simulink model "CartesianImpedanceCtrlForUse"  (R2024a)
settings: Solver=ode45  StartTime=0.0  StopTime=tEnd+7  RelTol=1e-3
values from neighbouring files (symbols this model uses):
  Kf_gain = 100    [helperDesignImpedanceControl.m]
  neuromeka = importrobot(robotFile, DataFormat="column")    [helperDesignImpedanceControl.m]
  objectPos = 0.2    [helperDesignImpedanceControl.m]
  p_surface = [-0.30; -0.20; 0.35]    [helperDesignImpedanceControl.m]
  q_init = q_nmpc    [helperDesignImpedanceControl.m]
  tEnd = 5    [helperDesignImpedanceControl.m]
  Ts = 0.001    [helperDesignImpedanceControl.m]
  tStart = 0.5    [helperDesignImpedanceControl.m]
  use_force_feedback = 1    [helperDesignImpedanceControl.m]
undefined symbols (not defined in the file or in its folder): X, Y, Z
libraries: sm_lib x88, nesl_utility x54, matrix_library x4, robotcorelib x2, robotmaniplib x2, simulink x1
(part 3 of 3)

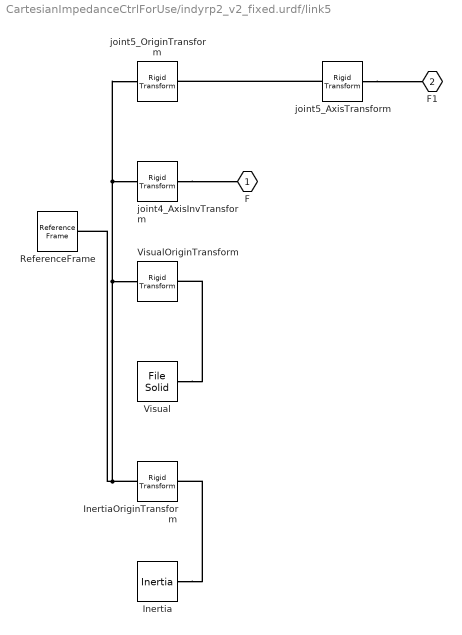
== system CartesianImpedanceCtrlForUse/indyrp2_v2_fixed.urdf/link5 ==
  Inertia : sm_lib/Body Elements/Inertia  InertiaType=Custom  Mass=2.12830848  MassUnits=kg  CenterOfMass=[0, 0, 0]  CenterOfMassUnits=m  MomentsOfInertia=[0.02795227, 0.0143985, 0.01495514]  MomentsOfInertiaUnits=kg*m^2  ProductsOfInertia=[-0.01265087, -4.713e-05, 3.938e-05]  ProductsOfInertiaUnits=kg*m^2  GraphicType=None  MarkerShape=Inertia  MarkerSize=20  GraphicVisPropType=SimpleVisualProperties  GraphicDiffuseColor=[0.5 0.5 0.5]  GraphicOpacity=1  GraphicSpecularColor=[0.5 0.5 0.5 1.0]  GraphicAmbientColor=[0.15 0.15 0.15 1.0]  GraphicEmissiveColor=[0.0 0.0 0.0 1.0]  GraphicShininess=75
  InertiaOriginTransform : sm_lib/Frames and Transforms/Rigid Transform  RotationMethod=RotationSequence  FollAlignAxisA=+X  BaseAlignAxisA=+Y  FollAlignAxisB=+Y  BaseAlignAxisB=+Z  RotationStandardAxis=+Z  RotationAngle=0  RotationAngleUnits=deg  RotationArbitraryAxis=[0 0 1]  RotationSequenceAxes=BaseAxes  RotationSequence=XYZ  RotationSequenceAngles=[0, 0, 0]  RotationSequenceAnglesUnits=rad  RotationMatrix=[1 0 0;0 1 0;0 0 1]  Quaternion=[1 0 0 0]  TranslationMethod=Cartesian  TranslationCartesianOffset=[-0.00026808, -0.07105971, 0.07645328999999999]  TranslationCartesianOffsetUnits=m  TranslationStandardAxis=+Z  TranslationStandardOffset=0  TranslationStandardOffsetUnits=m  TranslationROffset=0  TranslationROffsetUnits=m  TranslationThetaOffset=0  TranslationThetaOffsetUnits=deg  TranslationZOffset=0  TranslationZOffsetUnits=m
  ReferenceFrame : sm_lib/Frames and Transforms/Reference Frame
  Visual : sm_lib/Body Elements/File Solid  ExtGeomFileName=../meshes/indyrp2_v2/visual/IndyRP2_v2_5.stl  UnitType=Custom  ExtGeomFileUnits=m  StepReaderType=HEX  ExportConvexHullGeometry=off  InertiaType=Custom  BasedOnType=DensityFromFile  Density=1000  DensityUnits=kg/m^3  Mass=0  MassUnits=kg  CenterOfMass=[0, 0, 0]  CenterOfMassUnits=m  MomentsOfInertia=[0, 0, 0]  MomentsOfInertiaUnits=kg*m^2  ProductsOfInertia=[0, 0, 0]  ProductsOfInertiaUnits=kg*m^2  GraphicType=FromGeometry  MarkerShape=Sphere  MarkerSize=10  GraphicVisPropType=SimpleVisualProperties  GraphicDiffuseColor=[0.8941176470588236, 0.8941176470588236, 0.8941176470588236]  GraphicOpacity=1  GraphicSpecularColor=[0.5 0.5 0.5 1.0]  GraphicAmbientColor=[0.15 0.15 0.15 1.0]  GraphicEmissiveColor=[0.0 0.0 0.0 1.0]  GraphicShininess=75  DoExposeReferenceFrame=on  SerializedFrames=<Frames/>
  VisualOriginTransform : sm_lib/Frames and Transforms/Rigid Transform  RotationMethod=RotationSequence  FollAlignAxisA=+X  BaseAlignAxisA=+Y  FollAlignAxisB=+Y  BaseAlignAxisB=+Z  RotationStandardAxis=+Z  RotationAngle=0  RotationAngleUnits=deg  RotationArbitraryAxis=[0 0 1]  RotationSequenceAxes=BaseAxes  RotationSequence=XYZ  RotationSequenceAngles=[0, 0, 0]  RotationSequenceAnglesUnits=rad  RotationMatrix=[1 0 0;0 1 0;0 0 1]  Quaternion=[1 0 0 0]  TranslationMethod=Cartesian  TranslationCartesianOffset=[0, 0, 0]  TranslationCartesianOffsetUnits=m  TranslationStandardAxis=+Z  TranslationStandardOffset=0  TranslationStandardOffsetUnits=m  TranslationROffset=0  TranslationROffsetUnits=m  TranslationThetaOffset=0  TranslationThetaOffsetUnits=deg  TranslationZOffset=0  TranslationZOffsetUnits=m
  joint4_AxisInvTransform : sm_lib/Frames and Transforms/Rigid Transform  RotationMethod=ArbitraryAxis  FollAlignAxisA=+X  BaseAlignAxisA=+Y  FollAlignAxisB=+Y  BaseAlignAxisB=+Z  RotationStandardAxis=+Z  RotationAngle=0  RotationAngleUnits=rad  RotationArbitraryAxis=[1, 0, 0]  RotationSequenceAxes=FollowerAxes  RotationSequence=XYX  RotationSequenceAngles=[0 0 0]  RotationSequenceAnglesUnits=deg  RotationMatrix=[1 0 0;0 1 0;0 0 1]  Quaternion=[1 0 0 0]  TranslationMethod=Cartesian  TranslationCartesianOffset=[0, 0, 0]  TranslationCartesianOffsetUnits=m  TranslationStandardAxis=+Z  TranslationStandardOffset=0  TranslationStandardOffsetUnits=m  TranslationROffset=0  TranslationROffsetUnits=m  TranslationThetaOffset=0  TranslationThetaOffsetUnits=deg  TranslationZOffset=0  TranslationZOffsetUnits=m
  joint5_AxisTransform : sm_lib/Frames and Transforms/Rigid Transform  RotationMethod=ArbitraryAxis  FollAlignAxisA=+X  BaseAlignAxisA=+Y  FollAlignAxisB=+Y  BaseAlignAxisB=+Z  RotationStandardAxis=+Z  RotationAngle=0  RotationAngleUnits=rad  RotationArbitraryAxis=[1, 0, 0]  RotationSequenceAxes=FollowerAxes  RotationSequence=XYX  RotationSequenceAngles=[0 0 0]  RotationSequenceAnglesUnits=deg  RotationMatrix=[1 0 0;0 1 0;0 0 1]  Quaternion=[1 0 0 0]  TranslationMethod=Cartesian  TranslationCartesianOffset=[0, 0, 0]  TranslationCartesianOffsetUnits=m  TranslationStandardAxis=+Z  TranslationStandardOffset=0  TranslationStandardOffsetUnits=m  TranslationROffset=0  TranslationROffsetUnits=m  TranslationThetaOffset=0  TranslationThetaOffsetUnits=deg  TranslationZOffset=0  TranslationZOffsetUnits=m
  joint5_OriginTransform : sm_lib/Frames and Transforms/Rigid Transform  RotationMethod=RotationSequence  FollAlignAxisA=+X  BaseAlignAxisA=+Y  FollAlignAxisB=+Y  BaseAlignAxisB=+Z  RotationStandardAxis=+Z  RotationAngle=0  RotationAngleUnits=deg  RotationArbitraryAxis=[0 0 1]  RotationSequenceAxes=BaseAxes  RotationSequence=XYZ  RotationSequenceAngles=[1.570796327, 0, 0]  RotationSequenceAnglesUnits=rad  RotationMatrix=[1 0 0;0 1 0;0 0 1]  Quaternion=[1 0 0 0]  TranslationMethod=Cartesian  TranslationCartesianOffset=[0, -0.114, 0.0835]  TranslationCartesianOffsetUnits=m  TranslationStandardAxis=+Z  TranslationStandardOffset=0  TranslationStandardOffsetUnits=m  TranslationROffset=0  TranslationROffsetUnits=m  TranslationThetaOffset=0  TranslationThetaOffsetUnits=deg  TranslationZOffset=0  TranslationZOffsetUnits=m
  F : PMIOPort  Side=Left
  F1 : PMIOPort  Port=2  Side=Right
  connections:
  Inertia/RConn1 -- InertiaOriginTransform/RConn1
  InertiaOriginTransform/LConn1 -- joint4_AxisInvTransform/LConn1 -- joint5_OriginTransform/LConn1 -- VisualOriginTransform/LConn1 -- ReferenceFrame/RConn1
  Visual/RConn1 -- VisualOriginTransform/RConn1
  joint4_AxisInvTransform/RConn1 -- F/RConn1
  joint5_AxisTransform/RConn1 -- F1/RConn1
  joint5_AxisTransform/LConn1 -- joint5_OriginTransform/RConn1

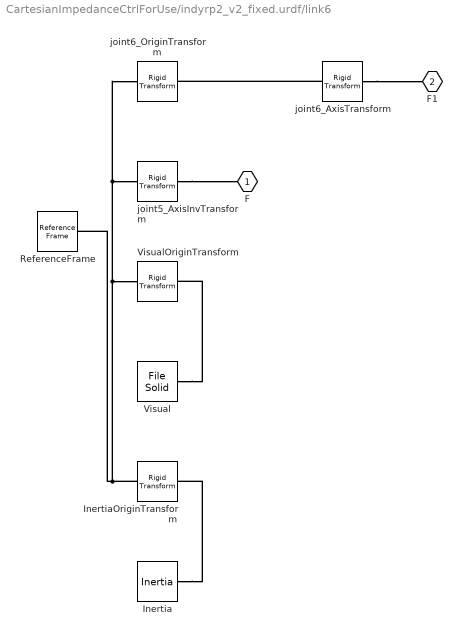
== system CartesianImpedanceCtrlForUse/indyrp2_v2_fixed.urdf/link6 ==
  Inertia : sm_lib/Body Elements/Inertia  InertiaType=Custom  Mass=2.32413397  MassUnits=kg  CenterOfMass=[0, 0, 0]  CenterOfMassUnits=m  MomentsOfInertia=[0.01771876, 0.01593616, 0.00358348]  MomentsOfInertiaUnits=kg*m^2  ProductsOfInertia=[-0.00069656, -4.336e-05, 9.04e-06]  ProductsOfInertiaUnits=kg*m^2  GraphicType=None  MarkerShape=Inertia  MarkerSize=20  GraphicVisPropType=SimpleVisualProperties  GraphicDiffuseColor=[0.5 0.5 0.5]  GraphicOpacity=1  GraphicSpecularColor=[0.5 0.5 0.5 1.0]  GraphicAmbientColor=[0.15 0.15 0.15 1.0]  GraphicEmissiveColor=[0.0 0.0 0.0 1.0]  GraphicShininess=75
  InertiaOriginTransform : sm_lib/Frames and Transforms/Rigid Transform  RotationMethod=RotationSequence  FollAlignAxisA=+X  BaseAlignAxisA=+Y  FollAlignAxisB=+Y  BaseAlignAxisB=+Z  RotationStandardAxis=+Z  RotationAngle=0  RotationAngleUnits=deg  RotationArbitraryAxis=[0 0 1]  RotationSequenceAxes=BaseAxes  RotationSequence=XYZ  RotationSequenceAngles=[0, 0, 0]  RotationSequenceAnglesUnits=rad  RotationMatrix=[1 0 0;0 1 0;0 0 1]  Quaternion=[1 0 0 0]  TranslationMethod=Cartesian  TranslationCartesianOffset=[-0.00022538, -0.00354123, 0.07650762]  TranslationCartesianOffsetUnits=m  TranslationStandardAxis=+Z  TranslationStandardOffset=0  TranslationStandardOffsetUnits=m  TranslationROffset=0  TranslationROffsetUnits=m  TranslationThetaOffset=0  TranslationThetaOffsetUnits=deg  TranslationZOffset=0  TranslationZOffsetUnits=m
  ReferenceFrame : sm_lib/Frames and Transforms/Reference Frame
  Visual : sm_lib/Body Elements/File Solid  ExtGeomFileName=../meshes/indyrp2_v2/visual/IndyRP2_v2_6.stl  UnitType=Custom  ExtGeomFileUnits=m  StepReaderType=HEX  ExportConvexHullGeometry=off  InertiaType=Custom  BasedOnType=DensityFromFile  Density=1000  DensityUnits=kg/m^3  Mass=0  MassUnits=kg  CenterOfMass=[0, 0, 0]  CenterOfMassUnits=m  MomentsOfInertia=[0, 0, 0]  MomentsOfInertiaUnits=kg*m^2  ProductsOfInertia=[0, 0, 0]  ProductsOfInertiaUnits=kg*m^2  GraphicType=FromGeometry  MarkerShape=Sphere  MarkerSize=10  GraphicVisPropType=SimpleVisualProperties  GraphicDiffuseColor=[0.8941176470588236, 0.8941176470588236, 0.8941176470588236]  GraphicOpacity=1  GraphicSpecularColor=[0.5 0.5 0.5 1.0]  GraphicAmbientColor=[0.15 0.15 0.15 1.0]  GraphicEmissiveColor=[0.0 0.0 0.0 1.0]  GraphicShininess=75  DoExposeReferenceFrame=on  SerializedFrames=<Frames/>
  VisualOriginTransform : sm_lib/Frames and Transforms/Rigid Transform  RotationMethod=RotationSequence  FollAlignAxisA=+X  BaseAlignAxisA=+Y  FollAlignAxisB=+Y  BaseAlignAxisB=+Z  RotationStandardAxis=+Z  RotationAngle=0  RotationAngleUnits=deg  RotationArbitraryAxis=[0 0 1]  RotationSequenceAxes=BaseAxes  RotationSequence=XYZ  RotationSequenceAngles=[0, 0, 0]  RotationSequenceAnglesUnits=rad  RotationMatrix=[1 0 0;0 1 0;0 0 1]  Quaternion=[1 0 0 0]  TranslationMethod=Cartesian  TranslationCartesianOffset=[0, 0, 0]  TranslationCartesianOffsetUnits=m  TranslationStandardAxis=+Z  TranslationStandardOffset=0  TranslationStandardOffsetUnits=m  TranslationROffset=0  TranslationROffsetUnits=m  TranslationThetaOffset=0  TranslationThetaOffsetUnits=deg  TranslationZOffset=0  TranslationZOffsetUnits=m
  joint5_AxisInvTransform : sm_lib/Frames and Transforms/Rigid Transform  RotationMethod=ArbitraryAxis  FollAlignAxisA=+X  BaseAlignAxisA=+Y  FollAlignAxisB=+Y  BaseAlignAxisB=+Z  RotationStandardAxis=+Z  RotationAngle=0  RotationAngleUnits=rad  RotationArbitraryAxis=[1, 0, 0]  RotationSequenceAxes=FollowerAxes  RotationSequence=XYX  RotationSequenceAngles=[0 0 0]  RotationSequenceAnglesUnits=deg  RotationMatrix=[1 0 0;0 1 0;0 0 1]  Quaternion=[1 0 0 0]  TranslationMethod=Cartesian  TranslationCartesianOffset=[0, 0, 0]  TranslationCartesianOffsetUnits=m  TranslationStandardAxis=+Z  TranslationStandardOffset=0  TranslationStandardOffsetUnits=m  TranslationROffset=0  TranslationROffsetUnits=m  TranslationThetaOffset=0  TranslationThetaOffsetUnits=deg  TranslationZOffset=0  TranslationZOffsetUnits=m
  joint6_AxisTransform : sm_lib/Frames and Transforms/Rigid Transform  RotationMethod=ArbitraryAxis  FollAlignAxisA=+X  BaseAlignAxisA=+Y  FollAlignAxisB=+Y  BaseAlignAxisB=+Z  RotationStandardAxis=+Z  RotationAngle=0  RotationAngleUnits=rad  RotationArbitraryAxis=[1, 0, 0]  RotationSequenceAxes=FollowerAxes  RotationSequence=XYX  RotationSequenceAngles=[0 0 0]  RotationSequenceAnglesUnits=deg  RotationMatrix=[1 0 0;0 1 0;0 0 1]  Quaternion=[1 0 0 0]  TranslationMethod=Cartesian  TranslationCartesianOffset=[0, 0, 0]  TranslationCartesianOffsetUnits=m  TranslationStandardAxis=+Z  TranslationStandardOffset=0  TranslationStandardOffsetUnits=m  TranslationROffset=0  TranslationROffsetUnits=m  TranslationThetaOffset=0  TranslationThetaOffsetUnits=deg  TranslationZOffset=0  TranslationZOffsetUnits=m
  joint6_OriginTransform : sm_lib/Frames and Transforms/Rigid Transform  RotationMethod=RotationSequence  FollAlignAxisA=+X  BaseAlignAxisA=+Y  FollAlignAxisB=+Y  BaseAlignAxisB=+Z  RotationStandardAxis=+Z  RotationAngle=0  RotationAngleUnits=deg  RotationArbitraryAxis=[0 0 1]  RotationSequenceAxes=BaseAxes  RotationSequence=XYZ  RotationSequenceAngles=[-1.570796327, 0, 0]  RotationSequenceAnglesUnits=rad  RotationMatrix=[1 0 0;0 1 0;0 0 1]  Quaternion=[1 0 0 0]  TranslationMethod=Cartesian  TranslationCartesianOffset=[0, 0.052, 0.08500000000000001]  TranslationCartesianOffsetUnits=m  TranslationStandardAxis=+Z  TranslationStandardOffset=0  TranslationStandardOffsetUnits=m  TranslationROffset=0  TranslationROffsetUnits=m  TranslationThetaOffset=0  TranslationThetaOffsetUnits=deg  TranslationZOffset=0  TranslationZOffsetUnits=m
  F : PMIOPort  Side=Left
  F1 : PMIOPort  Port=2  Side=Right
  connections:
  Inertia/RConn1 -- InertiaOriginTransform/RConn1
  InertiaOriginTransform/LConn1 -- joint5_AxisInvTransform/LConn1 -- joint6_OriginTransform/LConn1 -- VisualOriginTransform/LConn1 -- ReferenceFrame/RConn1
  Visual/RConn1 -- VisualOriginTransform/RConn1
  joint5_AxisInvTransform/RConn1 -- F/RConn1
  joint6_AxisTransform/RConn1 -- F1/RConn1
  joint6_AxisTransform/LConn1 -- joint6_OriginTransform/RConn1

== system CartesianImpedanceCtrlForUse/indyrp2_v2_fixed.urdf/link7 ==
  Inertia : sm_lib/Body Elements/Inertia  InertiaType=Custom  Mass=0.39652271  MassUnits=kg  CenterOfMass=[0, 0, 0]  CenterOfMassUnits=m  MomentsOfInertia=[0.00077839, 0.00076561, 0.00051275]  MomentsOfInertiaUnits=kg*m^2  ProductsOfInertia=[-6.99e-06, 0, 2.6e-07]  ProductsOfInertiaUnits=kg*m^2  GraphicType=None  MarkerShape=Inertia  MarkerSize=20  GraphicVisPropType=SimpleVisualProperties  GraphicDiffuseColor=[0.5 0.5 0.5]  GraphicOpacity=1  GraphicSpecularColor=[0.5 0.5 0.5 1.0]  GraphicAmbientColor=[0.15 0.15 0.15 1.0]  GraphicEmissiveColor=[0.0 0.0 0.0 1.0]  GraphicShininess=75
  InertiaOriginTransform : sm_lib/Frames and Transforms/Rigid Transform  RotationMethod=RotationSequence  FollAlignAxisA=+X  BaseAlignAxisA=+Y  FollAlignAxisB=+Y  BaseAlignAxisB=+Z  RotationStandardAxis=+Z  RotationAngle=0  RotationAngleUnits=deg  RotationArbitraryAxis=[0 0 1]  RotationSequenceAxes=BaseAxes  RotationSequence=XYZ  RotationSequenceAngles=[0, 0, 0]  RotationSequenceAnglesUnits=rad  RotationMatrix=[1 0 0;0 1 0;0 0 1]  Quaternion=[1 0 0 0]  TranslationMethod=Cartesian  TranslationCartesianOffset=[0, -0.00071501, 0.03219123]  TranslationCartesianOffsetUnits=m  TranslationStandardAxis=+Z  TranslationStandardOffset=0  TranslationStandardOffsetUnits=m  TranslationROffset=0  TranslationROffsetUnits=m  TranslationThetaOffset=0  TranslationThetaOffsetUnits=deg  TranslationZOffset=0  TranslationZOffsetUnits=m
  ReferenceFrame : sm_lib/Frames and Transforms/Reference Frame
  Visual : sm_lib/Body Elements/File Solid  ExtGeomFileName=../meshes/indyrp2_v2/visual/IndyRP2_v2_7.stl  UnitType=Custom  ExtGeomFileUnits=m  StepReaderType=HEX  ExportConvexHullGeometry=off  InertiaType=Custom  BasedOnType=DensityFromFile  Density=1000  DensityUnits=kg/m^3  Mass=0  MassUnits=kg  CenterOfMass=[0, 0, 0]  CenterOfMassUnits=m  MomentsOfInertia=[0, 0, 0]  MomentsOfInertiaUnits=kg*m^2  ProductsOfInertia=[0, 0, 0]  ProductsOfInertiaUnits=kg*m^2  GraphicType=FromGeometry  MarkerShape=Sphere  MarkerSize=10  GraphicVisPropType=SimpleVisualProperties  GraphicDiffuseColor=[0.8941176470588236, 0.8941176470588236, 0.8941176470588236]  GraphicOpacity=1  GraphicSpecularColor=[0.5 0.5 0.5 1.0]  GraphicAmbientColor=[0.15 0.15 0.15 1.0]  GraphicEmissiveColor=[0.0 0.0 0.0 1.0]  GraphicShininess=75  DoExposeReferenceFrame=on  SerializedFrames=<Frames/>
  VisualOriginTransform : sm_lib/Frames and Transforms/Rigid Transform  RotationMethod=RotationSequence  FollAlignAxisA=+X  BaseAlignAxisA=+Y  FollAlignAxisB=+Y  BaseAlignAxisB=+Z  RotationStandardAxis=+Z  RotationAngle=0  RotationAngleUnits=deg  RotationArbitraryAxis=[0 0 1]  RotationSequenceAxes=BaseAxes  RotationSequence=XYZ  RotationSequenceAngles=[0, 0, 0]  RotationSequenceAnglesUnits=rad  RotationMatrix=[1 0 0;0 1 0;0 0 1]  Quaternion=[1 0 0 0]  TranslationMethod=Cartesian  TranslationCartesianOffset=[0, 0, 0]  TranslationCartesianOffsetUnits=m  TranslationStandardAxis=+Z  TranslationStandardOffset=0  TranslationStandardOffsetUnits=m  TranslationROffset=0  TranslationROffsetUnits=m  TranslationThetaOffset=0  TranslationThetaOffsetUnits=deg  TranslationZOffset=0  TranslationZOffsetUnits=m
  joint6_AxisInvTransform : sm_lib/Frames and Transforms/Rigid Transform  RotationMethod=ArbitraryAxis  FollAlignAxisA=+X  BaseAlignAxisA=+Y  FollAlignAxisB=+Y  BaseAlignAxisB=+Z  RotationStandardAxis=+Z  RotationAngle=0  RotationAngleUnits=rad  RotationArbitraryAxis=[1, 0, 0]  RotationSequenceAxes=FollowerAxes  RotationSequence=XYX  RotationSequenceAngles=[0 0 0]  RotationSequenceAnglesUnits=deg  RotationMatrix=[1 0 0;0 1 0;0 0 1]  Quaternion=[1 0 0 0]  TranslationMethod=Cartesian  TranslationCartesianOffset=[0, 0, 0]  TranslationCartesianOffsetUnits=m  TranslationStandardAxis=+Z  TranslationStandardOffset=0  TranslationStandardOffsetUnits=m  TranslationROffset=0  TranslationROffsetUnits=m  TranslationThetaOffset=0  TranslationThetaOffsetUnits=deg  TranslationZOffset=0  TranslationZOffsetUnits=m
  tcp_OriginTransform : sm_lib/Frames and Transforms/Rigid Transform  RotationMethod=RotationSequence  FollAlignAxisA=+X  BaseAlignAxisA=+Y  FollAlignAxisB=+Y  BaseAlignAxisB=+Z  RotationStandardAxis=+Z  RotationAngle=0  RotationAngleUnits=deg  RotationArbitraryAxis=[0 0 1]  RotationSequenceAxes=BaseAxes  RotationSequence=XYZ  RotationSequenceAngles=[0, 0, 0]  RotationSequenceAnglesUnits=rad  RotationMatrix=[1 0 0;0 1 0;0 0 1]  Quaternion=[1 0 0 0]  TranslationMethod=Cartesian  TranslationCartesianOffset=[0, 0, 0.057]  TranslationCartesianOffsetUnits=m  TranslationStandardAxis=+Z  TranslationStandardOffset=0  TranslationStandardOffsetUnits=m  TranslationROffset=0  TranslationROffsetUnits=m  TranslationThetaOffset=0  TranslationThetaOffsetUnits=deg  TranslationZOffset=0  TranslationZOffsetUnits=m
  F : PMIOPort  Side=Left
  F1 : PMIOPort  Port=2  Side=Right
  connections:
  Inertia/RConn1 -- InertiaOriginTransform/RConn1
  InertiaOriginTransform/LConn1 -- joint6_AxisInvTransform/LConn1 -- tcp_OriginTransform/LConn1 -- VisualOriginTransform/LConn1 -- ReferenceFrame/RConn1
  Visual/RConn1 -- VisualOriginTransform/RConn1
  joint6_AxisInvTransform/RConn1 -- F/RConn1
  tcp_OriginTransform/RConn1 -- F1/RConn1

== system CartesianImpedanceCtrlForUse/ImpedanceController/SpatialSpringWrench/InvertH ==
  Hx0 : Inport
  Constant : Constant  Value=[0 0 0 1]  VectorParams1D=off
  Gain : Gain  Gain=-1
  Matrix Concatenate : Concatenate  Mode=Multidimensional array  ConcatenateDimension=2
  Matrix Concatenate1 : Concatenate  Mode=Multidimensional array
  Matrix Multiply : Product  Multiplication=Matrix(*)
  Submatrix : matrix_library/Submatrix  RowSpan=Range of rows  RowStartMode=First  RowStartIndex=1  RowEndMode=Index  RowEndIndex=3  ColSpan=Range of columns  ColStartMode=First  ColStartIndex=1  ColEndMode=Index  ColEndIndex=3
  Submatrix1 : matrix_library/Submatrix  RowSpan=Range of rows  RowStartMode=First  RowStartIndex=1  RowEndMode=Index  RowEndIndex=3  ColSpan=One column  ColStartMode=Last  ColStartIndex=1  ColEndMode=Index  ColEndIndex=3
  Transpose : Math  Operator=transpose
  H0x : Outport
  wires:
  Matrix Concatenate1/1 -> H0x/1
  Matrix Concatenate/1 -> Matrix Concatenate1/1
  Submatrix1/1 -> Matrix Multiply/2
  Matrix Multiply/1 -> Matrix Concatenate/2
  Gain/1 -> Matrix Multiply/1
  Submatrix/1 -> Transpose/1
  Constant/1 -> Matrix Concatenate1/2
  Hx0/1 -> Submatrix/1, Submatrix1/1
  Transpose/1 -> Gain/1, Matrix Concatenate/1

== system CartesianImpedanceCtrlForUse/ImpedanceController/SpatialSpringWrench/InvertH1 ==
  Hx0 : Inport
  Constant : Constant  Value=[0 0 0 1]  VectorParams1D=off
  Gain : Gain  Gain=-1
  Matrix Concatenate : Concatenate  Mode=Multidimensional array  ConcatenateDimension=2
  Matrix Concatenate1 : Concatenate  Mode=Multidimensional array
  Matrix Multiply : Product  Multiplication=Matrix(*)
  Submatrix : matrix_library/Submatrix  RowSpan=Range of rows  RowStartMode=First  RowStartIndex=1  RowEndMode=Index  RowEndIndex=3  ColSpan=Range of columns  ColStartMode=First  ColStartIndex=1  ColEndMode=Index  ColEndIndex=3
  Submatrix1 : matrix_library/Submatrix  RowSpan=Range of rows  RowStartMode=First  RowStartIndex=1  RowEndMode=Index  RowEndIndex=3  ColSpan=One column  ColStartMode=Last  ColStartIndex=1  ColEndMode=Index  ColEndIndex=3
  Transpose : Math  Operator=transpose
  H0x : Outport
  wires:
  Transpose/1 -> Matrix Concatenate/1, Gain/1
  Hx0/1 -> Submatrix1/1, Submatrix/1
  Constant/1 -> Matrix Concatenate1/2
  Submatrix/1 -> Transpose/1
  Gain/1 -> Matrix Multiply/1
  Matrix Multiply/1 -> Matrix Concatenate/2
  Submatrix1/1 -> Matrix Multiply/2
  Matrix Concatenate/1 -> Matrix Concatenate1/1
  Matrix Concatenate1/1 -> H0x/1

== matlab function CartesianImpedanceCtrlForUse/indyrp2_v2_fixed.urdf/Subsystem/MATLAB Function1 ==
  data: R input; T output; x input; y input; z input
function T = createHomTransMat(R,x,y,z)

T = eye(4);
T(1:3,1:3) = R;
T(1:3,4) = [x y z]';

== matlab function CartesianImpedanceCtrlForUse/indyrp2_v2_fixed.urdf/MATLAB Function ==
  data: vx input; dirVel output; vy input; vz input
function dirVel = findVelDirection(vx,vy,vz)

if norm([vx,vy,vz]) <= eps
    dirVel = [0 0 0];
else
    dirVel = [vx vy vz]/norm([vx,vy,vz]);
end
end

== matlab function CartesianImpedanceCtrlForUse/ImpedanceController/Force Controller ==
  data: F_measured input; tau_force output; F_desired input; Kf input; J input
function tau_force = forceController(F_measured, F_desired, Kf, J)
%#codegen
% Force feedback contribution to joint torques
% Wrench ordering: [Torque(3); Force(3)]

    % Force error
    dF = F_desired - F_measured;
    
    % Build 6x1 wrench correction (zero torque, force correction only)
    wrench_correction = [zeros(3,1); Kf * dF];
    
    % Map to joint space
    tau_force = J' * wrench_correction;
end

== matlab function CartesianImpedanceCtrlForUse/ImpedanceController/Screw Phase Manager ==
  data: F_measured input; F_desired output; t input; Kf_phase output; phase_out output; screw_depth output; screw_angle output; friction_torque output; debug_out output; enable_Kf input; Kf_value input
function [F_desired, Kf_phase, phase_out, screw_depth, screw_angle, friction_torque, debug_out] = ...
    screwPhaseManager(F_measured, t, enable_Kf, Kf_value)
    %#codegen

    %% Persistent state
    persistent current_phase t_phase_start cumulative_angle
    if isempty(current_phase)
        current_phase = 0;
        t_phase_start = 0;
        cumulative_angle = 0;
    end

    %% Physical parameters (ISO 261, Wang et al. 2022)
    pitch = 0.8e-3;
    d_s = 5e-3;
    screw_length = 20e-3;
    c_f = 0.2;

    %% Force targets (reduced from 20/30N to 10/15N for realistic screwdriving)
    F_engage = 10;              % [N] was 20N, reduced to match screwdriving literature
    F_snug = 15;                % [N] was 30N, reduced for realistic contact

    %% Completion torque threshold
    tau_nominal = 0.003;        % [Nm] keep original

    %% Transition thresholds
    F_contact_threshold = 0.5;
    F_engage_threshold = 1.0;
    t_stable_required = 0.3;

    %% Rotation rate
    omega_screw = 25 * 2 * pi / 4.0;

    %% Default outputs
    F_desired = [0; 0; 0];
    Kf_phase = diag([0, 0, 0]);
    phase_out = 0;
    screw_depth = 0;
    screw_angle = 0;
    friction_torque = 0;

    %% Controller timestep
    dt = 0.001;

    %% Measured signals
    F_axial = abs(F_measured(3));

    %% Friction torque (Wang et al. 2022, Eq. 11)
    friction_torque = c_f * d_s * F_axial;

    %% Screw state
    screw_angle = cumulative_angle;
    screw_depth = (pitch / (2 * pi)) * screw_angle;

    %% Phase transitions
    switch current_phase
        case 0
            if F_axial > F_contact_threshold
                current_phase = 1;
                t_phase_start = t;
            end
        case 1
            if enable_Kf > 0
                if F_axial > F_engage_threshold && (t - t_phase_start) > t_stable_required
                    current_phase = 2;
                    t_phase_start = t;
                end
            end
        case 2
            cumulative_angle = cumulative_angle + omega_screw * dt;
            if screw_depth >= screw_length
                current_phase = 3;
                t_phase_start = t;
            end
        case 3
            if friction_torque >= tau_nominal && (t - t_phase_start) > 0.2
                current_phase = 4;
                t_phase_start = t;
            end
        case 4
    end

    %% Update screw state
    screw_angle = cumulative_angle;
    screw_depth = (pitch / (2 * pi)) * screw_angle;

    %% Phase-dependent outputs
    switch current_phase
        case 0
            F_desired = [0; 0; 0];
            Kf_phase = diag([0, 0, 0]);
        case 1
            F_desired = [0; 0; -F_engage];
            Kf_phase = diag([0, 0, Kf_value * enable_Kf]);
        case 2
            F_desired = [0; 0; -F_engage];
            Kf_phase = diag([0, 0, Kf_value * enable_Kf]);
        case 3
            F_desired = [0; 0; -F_snug];
            Kf_phase = diag([0, 0, Kf_value * enable_Kf]);
        case 4
            F_desired = [0; 0; 0];
            Kf_phase = diag([0, 0, 0]);
    end

    debug_out = F_axial;
    phase_out = current_phase;
end

== matlab function CartesianImpedanceCtrlForUse/ImpedanceController/SpatialSpringWrench/Adjoint ==
  data: H input; AdjH output
function AdjH = fcn(H)
%#codegen
R = H(1:3,1:3);
P = H(1:3,4);
AdjH = [     R       zeros(3);
         Tilde(P)*R     R      ];

== matlab function CartesianImpedanceCtrlForUse/ImpedanceController/SpatialSpringWrench/WrenchAtTip (considers stiffness parameters defined in mask) ==
  data: Htd input; W output; Go input; Gt input; Gc input
function W = fcn(Htd, Go, Gt, Gc)
% Calculates End-Effector wrench
%#codegen

% Rotation
Rtd = Htd(1:3,1:3);
% Position
Ptd = Htd(1:3,4);
%Calculate the moment 
Mt = -2*SkSym(Go*Rtd) - SkSym(Gt*Rtd'*Tilde(Ptd)*Tilde(Ptd)*Rtd) - 2*SkSym(Gc*Tilde(Ptd)*Rtd);
M = UnTilde(Mt);
%Calculate the force
Ft = -Rtd'*SkSym(Gt*Tilde(Ptd))*Rtd - SkSym(Gt*Rtd'*Tilde(Ptd)*Rtd) - 2*SkSym(Gc*Rtd);
F = UnTilde(Ft);
% wrench
W = [M;F];

== matlab function CartesianImpedanceCtrlForUse/indyrp2_v2_fixed.urdf/MATLAB Function1 ==
  data: fn input; wrenchContact output; ft input; velDir input; T input
function wrenchContact = estimateEEWrench(fn,ft,velDir,T)
%#codegen

%%% Ff = Adj_Taf'*Fa
wrenchContact = calcAdjMatrix(T(1:3,1:3),T(1:3,4))'*[0 0 0 -fn ft*-velDir(2) ft*-velDir(3)]'; 

end

function adjMat = calcAdjMatrix(R,p)
%#codegen
    adjMat = [R zeros(3); calcSkewSymMatrix(p)*R R];
end

function skewSymMat = calcSkewSymMatrix(v)
%#codegen
    x = v(1); y = v(2); z = v(3);
    skewSymMat = [0 -z y ; z 0 -x;-y x 0];
end

== matlab function CartesianImpedanceCtrlForUse/indyrp2_v2_fixed.urdf/MATLAB Function2 ==
  data: t input; Fx output; Fy output; Fz output
function [Fx, Fy, Fz] = externalPush(t)
    if t > 10 && t < 15
        Fx = 40; Fy = 0; Fz = 0;
    else
        Fx = 0; Fy = 0; Fz = 0;
    end
end
